simulink model "ControlDePos"  (R2017a)
settings: Solver=FixedStepAuto  StartTime=0.0  StopTime=stop_time  FixedStep=step_sim  MaxStep=0.1  RelTol=1e-4  EnableMultiTasking=on
values from neighbouring files (symbols this model uses):
  Kp = [kp,kp]    [runSim.m]
  Kv = [kv,kv]    [runSim.m]
libraries: roblocks x7, simulink x3, dspmtrx3 x1
settings Model: Creator=Tomas  LastModifiedBy=Santi
settings DataIOCC: LimitDataPoints=on  SaveOutput=off  SaveTime=off
settings OptimizationCC: ExpressionDepthLimit=2147483647  LifeSpan=1
settings DebuggingCC: UnderspecifiedInitializationDetection=Classic  MergeDetectMultiDrivingBlocksExec=none  FcnCallInpInsideContextMsg=warning  AllowSymbolicDim=off  StateNameClashWarn=warning  SFUnexpectedBacktrackingDiag=warning  SFNoUnconditionalDefaultTransitionDiag=warning  SFExecutionAtInitializationDiag=none
settings GRTTargetCC: TargetLangStandard=C89/C90 (ANSI)  GeneratePreprocessorConditionals=Disable all  CombineOutputUpdateFcns=off  GRTInterface=on

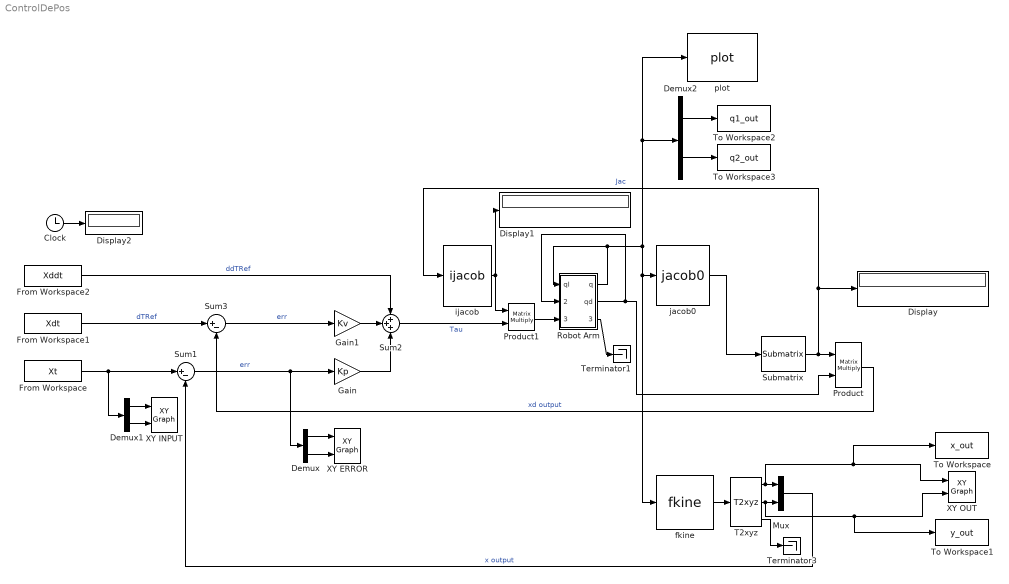
== system ControlDePos ==
  Clock : Clock
  Demux : Demux  Outputs=2
  Demux1 : Demux  Outputs=2
  Demux2 : Demux  Outputs=2
  Display : Display
  Display1 : Display
  Display2 : Display
  From Workspace : FromWorkspace  VariableName=Xt
  From Workspace1 : FromWorkspace  VariableName=Xdt
  From Workspace2 : FromWorkspace  VariableName=Xddt
  Gain : Gain  Gain=Kp
  Gain1 : Gain  Gain=Kv
  Mux : Mux  Inputs=2
  Product : Product  Multiplication=Matrix(*)
  Product1 : Product  Multiplication=Matrix(*)
  Robot Arm : Subsystem
  Submatrix : dspmtrx3/Submatrix  RowSpan=Range of rows  RowStartMode=First  RowStartIndex=1  RowEndMode=Index  RowEndIndex=2  ColSpan=Range of columns  ColStartMode=First  ColStartIndex=1  ColEndMode=Index  ColEndIndex=2
  Sum1 : Sum  Inputs=|+-
  Sum2 : Sum  Inputs=+++
  Sum3 : Sum  Inputs=|+-
  T2xyz : roblocks/Transform Conversion/T2xyz
  Terminator1 : Terminator
  Terminator3 : Terminator
  To Workspace : ToWorkspace  VariableName=x_out  SaveFormat=Timeseries  SampleTime=-1
  To Workspace1 : ToWorkspace  VariableName=y_out  SaveFormat=Timeseries  SampleTime=-1
  To Workspace2 : ToWorkspace  VariableName=q1_out  SaveFormat=Timeseries  SampleTime=-1
  To Workspace3 : ToWorkspace  VariableName=q2_out  SaveFormat=Timeseries  SampleTime=-1
  XY ERROR : simulink/Sinks/XY Graph  xmin=-2  xmax=2  ymin=-2  ymax=2  st=-1
  XY INPUT : simulink/Sinks/XY Graph  xmin=-2  xmax=2  ymin=-2  ymax=2  st=-1
  XY OUT : simulink/Sinks/XY Graph  xmin=-1  xmax=1  ymin=-1  ymax=1  st=-1
  fkine : roblocks/Kinematics/fkine  robot=wally
  ijacob : roblocks/Kinematics/ijacob
  "jacob0 " : roblocks/Kinematics/jacob0   robot=wally
  plot : roblocks/Robot Graphics/plot  robot=wally  fps=30  holdplot=on
      mask init:
      | %% Defino Plano.
      | p1 = [2 0 -2];
      | p2 = [0 2 -2];
      | p3 = [2 0  2];
      | p4 = [0 2  2];
      | 
      | points=[p1' p3' p4' p2'];
      | fill3(points(1,:),points(2,:),points(3,:),'r')
      | grid on
      | alpha(0.3)
  wires:
  Sum3/1 -> Gain1/1  "err"
  From Workspace1/1 -> Sum3/1  "dTRef"
  From Workspace2/1 -> Sum2/1  "ddTRef"
  Mux/1 -> Sum1/2  "x output"
  Sum1/1 -> Demux/1, Gain/1  "err"
  Product/1 -> Sum3/2  "xd output"
  Robot Arm/3(qdd) -> Terminator1/1
  fkine/1 -> T2xyz/1
  T2xyz/1 -> To Workspace/1, XY OUT/1, Mux/1
  T2xyz/2 -> To Workspace1/1, XY OUT/2, Mux/2
  T2xyz/3 -> Terminator3/1
  Robot Arm/2(qd) -> Product/2, Robot Arm/2(qdI)
  "jacob0 "/1 -> Submatrix/1
  Product1/1 -> Robot Arm/3(qddI)
  Robot Arm/1(q) -> Robot Arm/1(qI), Demux2/1, plot/1, fkine/1, "jacob0 "/1
  Gain/1 -> Sum2/3
  Gain1/1 -> Sum2/2
  Sum2/1 -> Product1/2  "Tau"
  ijacob/1 -> Display1/1, Product1/1
  Submatrix/1 -> Product/1, ijacob/1, Display/1  "Jac"
  Demux/1 -> XY ERROR/1
  Demux/2 -> XY ERROR/2
  Demux1/1 -> XY INPUT/1
  Demux1/2 -> XY INPUT/2
  Clock/1 -> Display2/1
  From Workspace/1 -> Sum1/1, Demux1/1
  Demux2/1 -> To Workspace2/1
  Demux2/2 -> To Workspace3/1

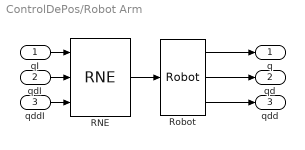
== system ControlDePos/Robot Arm ==
  qI : Inport
  qdI : Inport  Port=2
  qddI : Inport  Port=3
  RNE : roblocks/Dynamics/RNE  robot=wally  grav=[0 0 9.81]
  Robot : roblocks/Dynamics/Robot  robot=wally  q0=start_pos
  q : Outport
  qd : Outport  Port=2
  qdd : Outport  Port=3
  wires:
  qdI/1 -> RNE/2
  qI/1 -> RNE/1
  Robot/3 -> qdd/1
  Robot/1 -> q/1
  Robot/2 -> qd/1
  qddI/1 -> RNE/3
  RNE/1 -> Robot/1
